simulink model "example_2ofsum"  (R2021a)
settings: Solver=VariableStepAuto  StartTime=0.0  StopTime=1  RelTol=1e-3
settings Model: Creator=YasserNet  LastModifiedBy=YasserNet

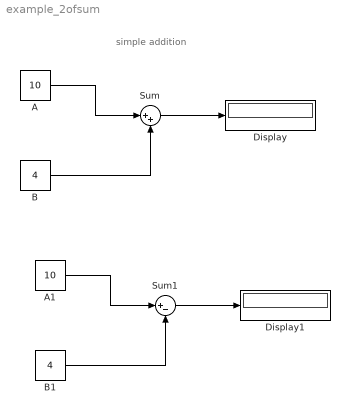
== system example_2ofsum ==
  note: simple addition
  A : Constant  Value=10
  A1 : Constant  Value=10
  B : Constant  Value=4
  B1 : Constant  Value=4
  Display : Display
  Display1 : Display
  Sum : Sum  Inputs=|++
  Sum1 : Sum  Inputs=|+-
  wires:
  A/1 -> Sum/1
  B/1 -> Sum/2
  Sum/1 -> Display/1
  A1/1 -> Sum1/1
  Sum1/1 -> Display1/1
  B1/1 -> Sum1/2
